simulink model "a_20210324_testahrs"  (R2020b)
settings: Solver=FixedStepAuto  StartTime=0.0  StopTime=inf  FixedStep=0.02  RelTol=1e-3  EnableMultiTasking=on
libraries: svdutilitieslib x2
settings Model: SILPILModeSetting=veronly  ExtModeBatchMode=on  ExtModeTrigDuration=2  Creator=ricca  LastModifiedBy=ricca
settings OptimizationCC: EnhancedBackFolding=on  PassReuseOutputArgsAs=Individual arguments  ZeroExternalMemoryAtStartup=off  ZeroInternalMemoryAtStartup=off  MaxStackSize=64  OptimizeBlockOrder=speed  DifferentSizesBufferReuse=on  OptimizationCustomize=off  EfficientTunableParamExpr=on
settings DebuggingCC: ParameterTunabilityLossMsg=error
settings HardwareCC: ProdBitPerPointer=32  ProdBitPerSizeT=32  ProdBitPerPtrDiffT=32  ProdLargestAtomicInteger=Long  ProdLargestAtomicFloat=Double  ProdEndianess=BigEndian  ProdWordSize=32  ProdHWDeviceType=ARM Compatible->ARM Cortex  UseEmbeddedCoderFeatures=off  UseSimulinkCoderFeatures=off
settings SFSimCC: MATLABDynamicMemAlloc=off
settings RTWCC: Description=Embedded Coder  SystemTargetFile=ert.tlc  HardwareBoard=Arduino Due  TemplateMakefile=ert_default_tmf  Toolchain=Arduino ARM  BuildConfiguration=Faster Runs
settings CodeAppCC: ForceParamTrailComments=on  IgnoreCustomStorageClasses=off  OperatorAnnotations=on  SimulinkDataObjDesc=on  SFDataObjDesc=on  MangleLength=10  InsertBlockDesc=on
settings ERTTargetCC: SupportContinuousTime=on  SupportNonInlinedSFcns=on  SupportVariableSizeSignals=on  ExtModeTransport=3  ExtModeStaticAllocSize=24576  ExtModeMexFile=ext_xcp  ExtModeIntrfLevel=Level2 - Open

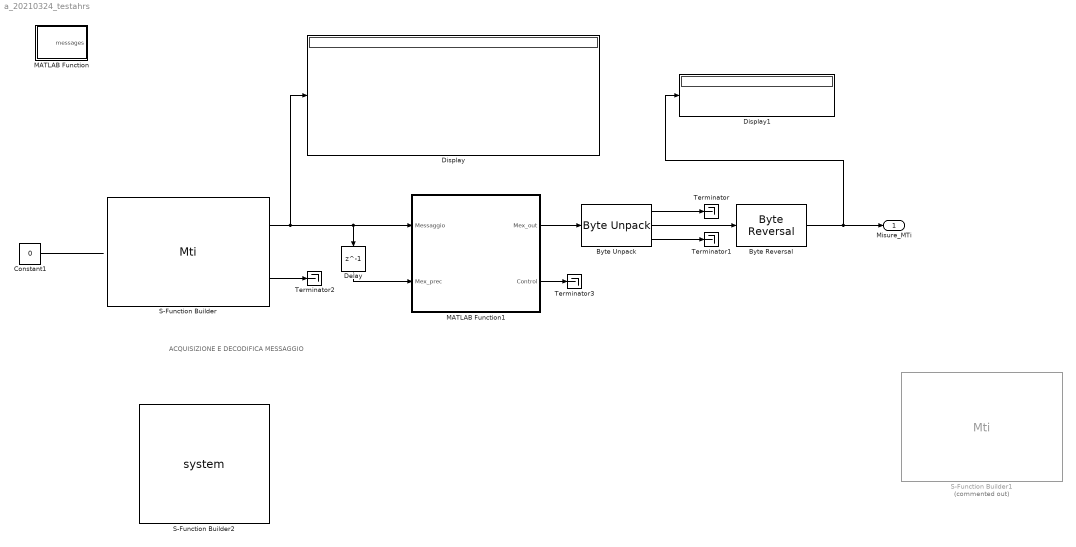
== system a_20210324_testahrs ==
  note: ACQUISIZIONE E DECODIFICA MESSAGGIO
  Byte Reversal : svdutilitieslib/Byte Reversal  numInp=1  blockPlatform=arduinoert
      settings: SourceProductBaseCode=ARDUINO
  Byte Unpack : svdutilitieslib/Byte Unpack  dimensions={[4],[9],[1]}  datatypes={'uint8','single','uint8'}  byteAlign=1  blockPlatform=arduinoert
      settings: SourceProductBaseCode=ARDUINO
  Constant1 : Constant  Value=0  OutDataTypeStr=uint8
  Delay : Delay  DelayLength=1
  Display : Display
  Display1 : Display
  MATLAB Function : MATLAB Function  TreatAsAtomicUnit=on
  MATLAB Function1 : MATLAB Function  TreatAsAtomicUnit=on
  S-Function Builder : S-Function  InitFcn=try, set_param(gcb,'FunctionName','Mti'), end  FunctionName=Mti  SFunctionModules=Mti_wrapper  SFunctionDeploymentMode=off  EnableBusSupport=off  mask(S-Function Builder){}
      mask help: Simulink:masks:SFunctionBuilder_MD
      mask init:
      | val = [[.9  0.75 0.75 1 1 .9 .9 1]',[1 1 0.75 0.75 .9 .9 1 .9]'];try , sys = get_param(gcb,'SfunBuilderFcnName');if isempty(sys), sys = get_param(gcb,'FunctionName'); end,catch, sys = get_param(gcb,'FunctionName'); end
      settings: CopyFcn=set_param(gcbh,'LinkStatus','none')  PreSaveFcn=try, set_param(gcb,'FunctionName','Mti'), end  OpenFcn=sfunctionwizard(gcbh)
      mask Display:
      | plot(val(:,1),val(:,2))
      | disp(sys)
      | port_label('input',1,'inutile')
      | port_label('output',1,'Messaggio')
      | port_label('output',2,'Control')
  S-Function Builder1 : S-Function  Commented=on  InitFcn=try, set_param(gcb,'FunctionName','Mti'), end  FunctionName=Mti  SFunctionModules=Mti_wrapper  SFunctionDeploymentMode=off  EnableBusSupport=off  mask(S-Function Builder){}
      mask help: Simulink:masks:SFunctionBuilder_MD
      mask init: same as a_20210324_testahrs/S-Function Builder
      settings: CopyFcn=set_param(gcbh,'LinkStatus','none')  PreSaveFcn=try, set_param(gcb,'FunctionName','Mti'), end  OpenFcn=sfunctionwizard(gcbh)
      mask Display:
      | plot(val(:,1),val(:,2))
      | disp(sys)
      | port_label('input',1,'inutile')
      | port_label('output',1,'Messaggio')
      | port_label('output',2,'Control')
  S-Function Builder2 : S-Function  SFunctionDeploymentMode=off  EnableBusSupport=off  mask(S-Function Builder){}
      mask help: Simulink:masks:SFunctionBuilder_MD
      mask init: same as a_20210324_testahrs/S-Function Builder
      settings: CopyFcn=set_param(gcbh,'LinkStatus','none')  OpenFcn=sfunctionwizard(gcbh)
      mask Display:
      | plot(val(:,1),val(:,2))
      | disp(sys)
  Terminator{,1..3} (4 alike) : Terminator
  Misure_MTi : Outport  VectorParamsAs1DForOutWhenUnconnected=off
  wires:
  Delay/1 -> MATLAB Function1/2(Mex_prec)
  Byte Unpack/3 -> Terminator1/1
  Byte Unpack/2 -> Byte Reversal/1
  MATLAB Function1/1(Mex_out) -> Byte Unpack/1
  MATLAB Function1/2(Control) -> Terminator3/1
  Byte Reversal/1 -> Display1/1, Misure_MTi/1
  S-Function Builder/2 -> Terminator2/1
  Constant1/1 -> ?
  Byte Unpack/1 -> Terminator/1
  S-Function Builder/1 -> Display/1, Delay/1, MATLAB Function1/1(Messaggio)

== matlab function a_20210324_testahrs/MATLAB Function1 ==
  data: Messaggio input; Mex_out output; Mex_prec input; Control output
function [Mex_out,Control]  = checksum_control(Messaggio,Mex_prec)

Control = uint8(0);

mti_string = uint8(Messaggio(2:41));

checksum = sum(mti_string) ; 

hex_checksum = dec2hex(checksum);

if ((hex_checksum(3) == '0') && (hex_checksum(4) == '0'))
    Mex_out = uint8(Messaggio);

else
   Control = uint8(1); 
   Mex_out = Mex_prec;   
end



end

== matlab function a_20210324_testahrs/MATLAB Function ==
  data: messages output
function messages =serialematlab
sett.port       = "COM5";
sett.baudrate	= 115200;
sett.byteorder	= "big-endian";

sett.SkipFactor             = 0xFFFF;                           % see pag. 41 of MT_Low_Level_Documentation.pdf
sett.header                 = 0xFA;
sett.ReqDID                 = [ 0xFA 0xFF 0x00 0x00 0x01 ];
sett.ReqOutputMode          = [ 0xFA 0xFF 0xD0 0x00 0x31 ];
sett.GoToMeasurement        = [ 0xFA 0xFF 0x10 0x00 0xF1 ];

% DA VERIFICARE IL CHECKSUM. I MESSAGGI SONO CISI' SCRITTI SONO INCORRETTI
% sett.ReqOutputSkipFactor    = [ 0xFA 0xFF 0xD4 0x00 0x01 ];     % see pag. 40 of MT_Low_Level_Documentation.pdf
% sett.ReqPortConfig          = [ 0xFA 0xFF 0x8C 0x00 0xE9 ];
% sett.WakeUp                 = [ 0xFA 0xFF 0x3E 0x00 0xE9 ];
% sett.GoToConfig             = [ 0xFA 0xFF 0x30 0x00 0xE9 ];
% sett.GoToMeasurement        = [ 0xFA 0xFF 0x10 0x00 0xE9 ];
% sett.ReqMTData              = [ ];

%%
fprintf( '\nApertura collegamento seriale su: %s -> ' , sett.port );
device = serialport( sett.port , sett.baudrate );
fprintf( '[ OK ]\n' );

%%
% see 5.1.1 Big endian output format on pag. 14 of MT_Low_Level_Documentation.pdf
fprintf( 'Imposto il ByteOrder a: %s -> ' , sett.byteorder );
device.ByteOrder = sett.byteorder;
fprintf( '[ OK ]\n\n' );
disp( device )

%%
fprintf( 'Richiedo le misure: -> ' );
write( device , sett.GoToMeasurement , "uint8" );
fprintf( '[ OK ]\n\n' );
disp( device )

%%

% esempio di comunicazione
% write( device , sett.ReqDID , "uint8" );
pause( 1 );
if ( device.NumBytesAvailable > 0 )
    
    % recupera tutto il buffer
    sms = read( device , device.NumBytesAvailable , "uint8" );
    sms_conv = reshape( [ dec2hex( sms )' ; ...
        repmat( ';' , 1 , length(sms) ) ] , 1 , [] );
    headers = strfind( sms_conv , dec2hex( sett.header ) );
    
    messages = cell( length( headers ) - 2 , 1 );
    
    for k = 1 : 1 : length( headers ) - 2
        
        messages{ k , 1 } = sms_conv( headers( k ) : 1 : headers( k + 1 ) - 2 );
        
        tmp = split( messages{ end }( 13 : end - 3 ) , ';' )
        typecast( hex2dec( tmp( 1 : 4)' )' , 'single' ) 
%         % converto il tipo (DA VERIFIARE)
%         sms_conv = typecast( sms , 'single' );
%         disp( sms_conv )
    end
    
else
    fprintf( '\n\n***\nNESSUN BYTE RICEVUTO!!!\n***\n\n' )
    
end
messages
end
